simulink model "HybridMotorcycle_HighLevelOverview"  (R2013a)
settings: Solver=ode45  StartTime=0.0  StopTime=10.0  RelTol=1e-3
libraries: fl_lib x4
settings Model: Creator=Raymond  LastModifiedBy=Raymond

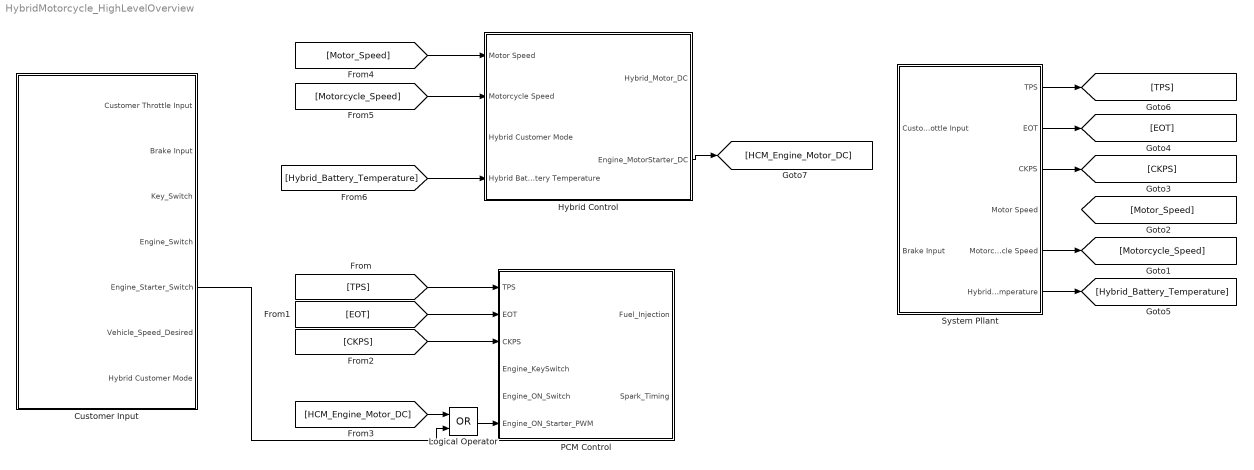
== system HybridMotorcycle_HighLevelOverview ==
  Customer Input : Subsystem
  Hybrid Control : Subsystem
  Logical Operator : Logic  Operator=OR  AllPortsSameDT=off  OutDataTypeStr=boolean
  PCM Control : Subsystem
  System Pllant : Subsystem
  wires:
  Customer Input/5(Engine_Starter_Switch) -> Logical Operator/2
  Logical Operator/1 -> PCM Control/6(Engine_ON_Starter_PWM)
  System Pllant/5(Motorcycle Speed) -> [Motorcycle_Speed]
  System Pllant/6(Hybrid Battery Temperature) -> [Hybrid_Battery_Temperature]
  System Pllant/1(TPS) -> [TPS]
  System Pllant/2(EOT) -> [EOT]
  System Pllant/3(CKPS) -> [CKPS]
  Hybrid Control/2(Engine_MotorStarter_DC) -> [HCM_Engine_Motor_DC]
  [TPS] -> PCM Control/1(TPS)
  [HCM_Engine_Motor_DC] -> Logical Operator/1
  [EOT] -> PCM Control/2(EOT)
  [CKPS] -> PCM Control/3(CKPS)
  [Motor_Speed] -> Hybrid Control/1(Motor Speed)
  [Motorcycle_Speed] -> Hybrid Control/2(Motorcycle Speed)
  [Hybrid_Battery_Temperature] -> Hybrid Control/4(Hybrid Battery Temperature)

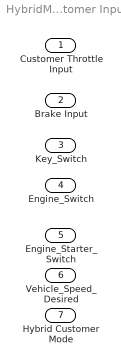
== system HybridMotorcycle_HighLevelOverview/Customer Input ==
  "Customer Throttle Input " : Outport
  Brake Input : Outport  Port=2
  Key_Switch : Outport  Port=3
  Engine_Switch : Outport  Port=4
  Engine_Starter_Switch : Outport  Port=5
  Vehicle_Speed_Desired : Outport  Port=6
  Hybrid Customer Mode : Outport  Port=7

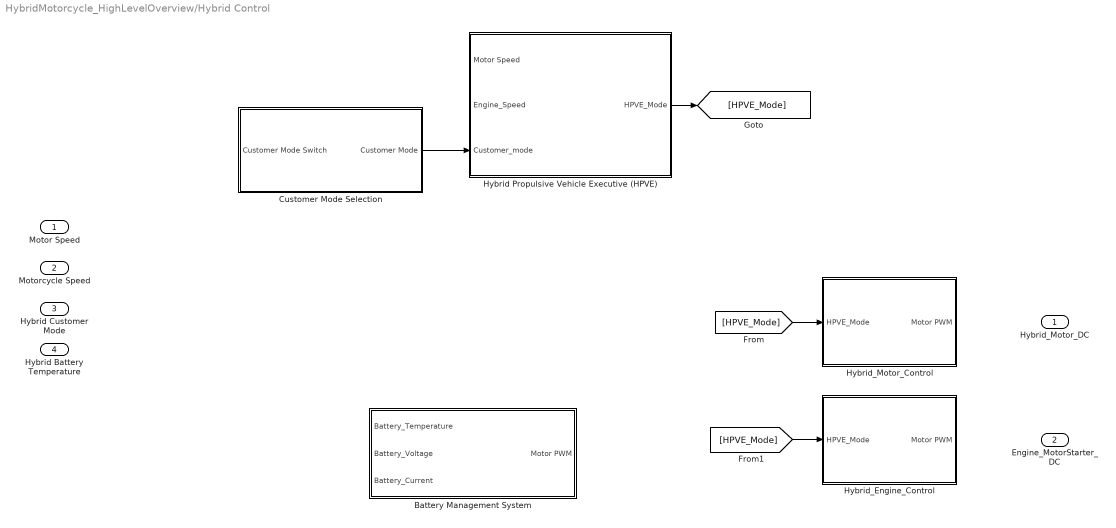
== system HybridMotorcycle_HighLevelOverview/Hybrid Control ==
  Motor Speed : Inport
  Motorcycle Speed : Inport  Port=2
  Hybrid Customer Mode : Inport  Port=3
  Hybrid Battery Temperature : Inport  Port=4
  Battery Management System : Subsystem
  Customer Mode Selection : Subsystem
  Hybrid Propulsive Vehicle Executive (HPVE) : Subsystem
  Hybrid_Engine_Control : Subsystem
  Hybrid_Motor_Control : Subsystem
  Hybrid_Motor_DC : Outport
  Engine_MotorStarter_DC : Outport  Port=2
  wires:
  [HPVE_Mode] -> Hybrid_Motor_Control/1(HPVE_Mode)
  [HPVE_Mode] -> Hybrid_Engine_Control/1(HPVE_Mode)
  Hybrid Propulsive Vehicle Executive (HPVE)/1(HPVE_Mode) -> [HPVE_Mode]
  Customer Mode Selection/1(Customer Mode) -> Hybrid Propulsive Vehicle Executive (HPVE)/3("Customer_mode ")

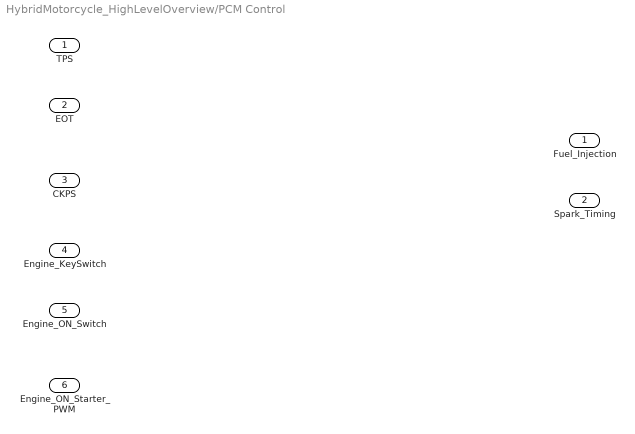
== system HybridMotorcycle_HighLevelOverview/PCM Control ==
  TPS : Inport
  EOT : Inport  Port=2
  CKPS : Inport  Port=3
  Engine_KeySwitch : Inport  Port=4
  Engine_ON_Switch : Inport  Port=5
  Engine_ON_Starter_PWM : Inport  Port=6
  Fuel_Injection : Outport
  Spark_Timing : Outport  Port=2

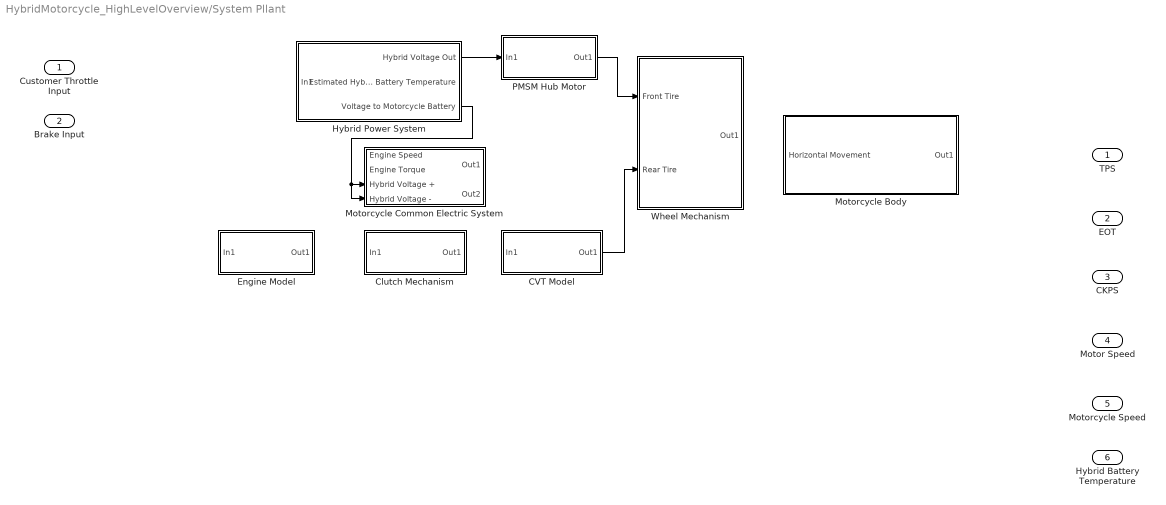
== system HybridMotorcycle_HighLevelOverview/System Pllant ==
  Customer Throttle Input : Inport
  Brake Input : Inport  Port=2
  CVT Model : Subsystem
  Clutch Mechanism : Subsystem
  Engine Model : Subsystem
  Hybrid Power System : Subsystem
  Motorcycle Body : Subsystem
  Motorcycle Common Electric System : Subsystem
  PMSM Hub Motor : Subsystem
  Wheel Mechanism : Subsystem
  TPS : Outport
  EOT : Outport  Port=2
  CKPS : Outport  Port=3
  Motor Speed : Outport  Port=4
  Motorcycle Speed : Outport  Port=5
  Hybrid Battery Temperature : Outport  Port=6
  wires:
  PMSM Hub Motor/1(Out1) -> Wheel Mechanism/1(Front Tire)
  CVT Model/1(Out1) -> Wheel Mechanism/2(Rear Tire)
  Hybrid Power System/1(Hybrid Voltage Out) -> PMSM Hub Motor/1(In1)
  Hybrid Power System/3(Voltage to Motorcycle Battery) -> Motorcycle Common Electric System/4(Hybrid Voltage -), Motorcycle Common Electric System/3(Hybrid Voltage +)

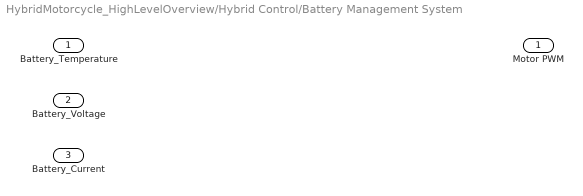
== system HybridMotorcycle_HighLevelOverview/Hybrid Control/Battery Management System ==
  Battery_Temperature : Inport
  Battery_Voltage : Inport  Port=2
  Battery_Current : Inport  Port=3
  Motor PWM : Outport

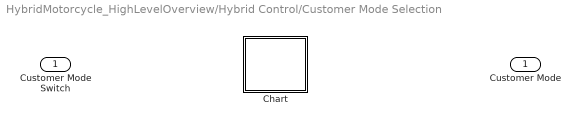
== system HybridMotorcycle_HighLevelOverview/Hybrid Control/Customer Mode Selection ==
  Customer Mode Switch : Inport
  Chart : Stateflow chart  TreatAsAtomicUnit=on
  Customer Mode : Outport

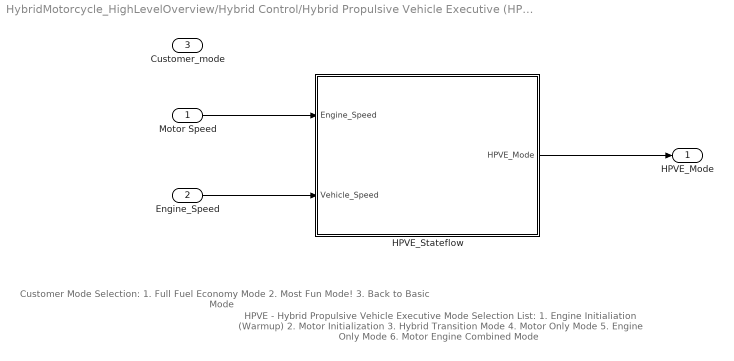
== system HybridMotorcycle_HighLevelOverview/Hybrid Control/Hybrid Propulsive Vehicle Executive (HPVE) ==
  note: Customer Mode Selection:
      |
      | 1. Full Fuel Economy Mode
      | 2. Most Fun Mode!
      | 3. Back to Basic Mode
  note: HPVE - Hybrid Propulsive Vehicle Executive
      | Mode Selection List:
      |
      | 1. Engine Initialiation (Warmup)
      | 2. Motor Initialization
      | 3. Hybrid Transition Mode
      | 4. Motor Only Mode
      | 5. Engine Only Mode
      | 6. Motor Engine Combined Mode
  Motor Speed : Inport
  Engine_Speed : Inport  Port=2
  "Customer_mode " : Inport  Port=3
  HPVE_Stateflow : Stateflow chart  TreatAsAtomicUnit=on
  HPVE_Mode : Outport
  wires:
  HPVE_Stateflow/1(HPVE_Mode) -> HPVE_Mode/1
  Motor Speed/1 -> HPVE_Stateflow/1(Engine_Speed)
  Engine_Speed/1 -> HPVE_Stateflow/2(Vehicle_Speed)

== system HybridMotorcycle_HighLevelOverview/Hybrid Control/Hybrid_Engine_Control ==
  HPVE_Mode : Inport
  Motor PWM : Outport

== system HybridMotorcycle_HighLevelOverview/Hybrid Control/Hybrid_Motor_Control ==
  HPVE_Mode : Inport
  Motor PWM : Outport

== system HybridMotorcycle_HighLevelOverview/System Pllant/CVT Model ==
  In1 : Inport
  Out1 : Outport
  wires:
  In1/1 -> Out1/1

== system HybridMotorcycle_HighLevelOverview/System Pllant/Clutch Mechanism ==
  In1 : Inport
  Out1 : Outport
  wires:
  In1/1 -> Out1/1

== system HybridMotorcycle_HighLevelOverview/System Pllant/Engine Model ==
  In1 : Inport
  Out1 : Outport
  wires:
  In1/1 -> Out1/1

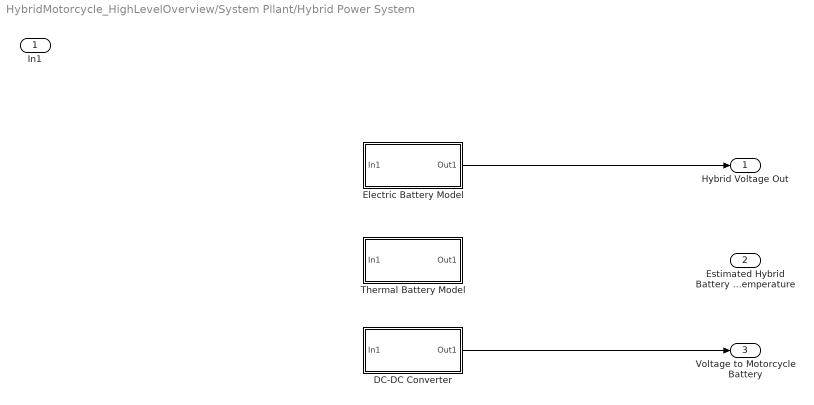
== system HybridMotorcycle_HighLevelOverview/System Pllant/Hybrid Power System ==
  In1 : Inport
  DC-DC Converter : Subsystem
  Electric Battery Model : Subsystem
  Thermal Battery Model : Subsystem
  Hybrid Voltage Out : Outport
  Estimated Hybrid Battery Temperature : Outport  Port=2
  Voltage to Motorcycle Battery : Outport  Port=3
  wires:
  DC-DC Converter/1(Out1) -> Voltage to Motorcycle Battery/1
  Electric Battery Model/1(Out1) -> Hybrid Voltage Out/1

== system HybridMotorcycle_HighLevelOverview/System Pllant/Motorcycle Body ==
  Horizontal Movement : Inport
  Out1 : Outport
  wires:
  Horizontal Movement/1 -> Out1/1

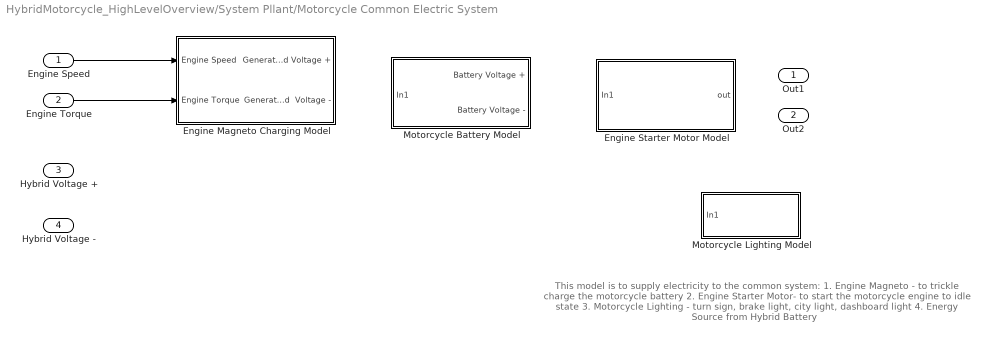
== system HybridMotorcycle_HighLevelOverview/System Pllant/Motorcycle Common Electric System ==
  note: This model is to supply electricity to the common system:
      | 1. Engine Magneto - to trickle charge the motorcycle battery
      | 2. Engine Starter Motor- to start the motorcycle engine to idle state
      | 3. Motorcycle Lighting - turn sign, brake light, city light, dashboard light
      | 4. Energy Source from Hybrid Battery
  Engine Speed : Inport
  Engine Torque : Inport  Port=2
  Hybrid Voltage + : Inport  Port=3
  Hybrid Voltage - : Inport  Port=4
  Engine Magneto Charging Model : Subsystem
  Engine Starter Motor Model : Subsystem
  Motorcycle Battery Model : Subsystem
  Motorcycle Lighting Model : Subsystem
  Out1 : Outport
  Out2 : Outport  Port=2
  wires:
  Engine Speed/1 -> Engine Magneto Charging Model/1(Engine Speed)
  Engine Torque/1 -> Engine Magneto Charging Model/2(Engine Torque)

== system HybridMotorcycle_HighLevelOverview/System Pllant/PMSM Hub Motor ==
  In1 : Inport
  Out1 : Outport
  wires:
  In1/1 -> Out1/1

== system HybridMotorcycle_HighLevelOverview/System Pllant/Wheel Mechanism ==
  Front Tire : Inport
  Rear Tire : Inport  Port=2
  Out1 : Outport
  wires:
  Front Tire/1 -> Out1/1

== system HybridMotorcycle_HighLevelOverview/System Pllant/Hybrid Power System/DC-DC Converter ==
  In1 : Inport
  Out1 : Outport
  wires:
  In1/1 -> Out1/1

== system HybridMotorcycle_HighLevelOverview/System Pllant/Hybrid Power System/Electric Battery Model ==
  In1 : Inport
  Out1 : Outport
  wires:
  In1/1 -> Out1/1

== system HybridMotorcycle_HighLevelOverview/System Pllant/Hybrid Power System/Thermal Battery Model ==
  In1 : Inport
  Out1 : Outport
  wires:
  In1/1 -> Out1/1

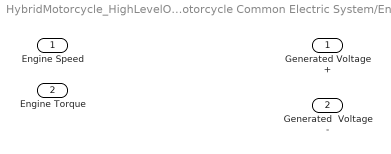
== system HybridMotorcycle_HighLevelOverview/System Pllant/Motorcycle Common Electric System/Engine Magneto Charging Model ==
  Engine Speed : Inport
  Engine Torque : Inport  Port=2
  Generated Voltage + : Outport
  Generated  Voltage - : Outport  Port=2

== system HybridMotorcycle_HighLevelOverview/System Pllant/Motorcycle Common Electric System/Engine Starter Motor Model ==
  In1 : Inport
  out : Outport

== system HybridMotorcycle_HighLevelOverview/System Pllant/Motorcycle Common Electric System/Motorcycle Battery Model ==
  In1 : Inport
  Battery Voltage + : Outport
  Battery Voltage - : Outport  Port=2

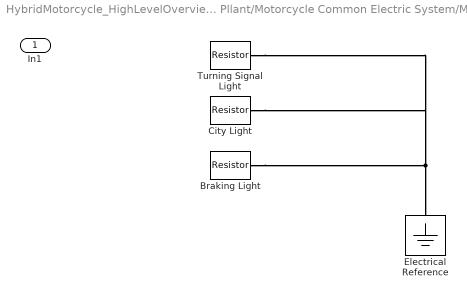
== system HybridMotorcycle_HighLevelOverview/System Pllant/Motorcycle Common Electric System/Motorcycle Lighting Model ==
  In1 : Inport
  Braking Light : fl_lib/Electrical/Electrical Elements/Resistor  R=1 Ohm  i_Log=off  v_Log=off  LocalVarNames=|i|v  LocalVarDescs=|i|v  LocalVarLogging=[0 0]
  City Light : fl_lib/Electrical/Electrical Elements/Resistor  R=1 Ohm  i_Log=off  v_Log=off  LocalVarNames=|i|v  LocalVarDescs=|i|v  LocalVarLogging=[0 0]
  Electrical Reference : fl_lib/Electrical/Electrical Elements/Electrical Reference  i_Log=off  LocalVarNames=|i  LocalVarDescs=|i  LocalVarLogging=0
  Turning Signal Light : fl_lib/Electrical/Electrical Elements/Resistor  R=1 Ohm  i_Log=off  v_Log=off  LocalVarNames=|i|v  LocalVarDescs=|i|v  LocalVarLogging=[0 0]
  connections:
  Braking Light/RConn1 -- Turning Signal Light/RConn1 -- City Light/RConn1 -- Electrical Reference/LConn1

== stateflow chart HybridMotorcycle_HighLevelOverview/Hybrid Control/Customer Mode Selection/Chart ==

== stateflow chart HybridMotorcycle_HighLevelOverview/Hybrid Control/Hybrid Propulsive Vehicle Executive (HPVE)/HPVE_Stateflow ==
  data: HPVE_Mode output double; Engine_Speed input double; Vehicle_Speed input double
